simulink model "sim2"  (R2015b)
settings: Solver=VariableStepAuto  StartTime=0.0  StopTime=50  RelTol=1e-3
values from neighbouring files (symbols this model uses):
  A1 = [0 1 0 ... (first row only)    [tp2.m]
  A2 = [0 1 0 ... (first row only)    [tp2.m]
  B1 = [0 ... (first row only)    [tp2.m]
  B2 = [0 ... (first row only)    [tp2.m]
  K1 = place(A1,B1,[lmb(1) lmb(2) 0])    [tp2.m]
  K2 = place(A2,B2,[lmb(1) lmb(2) 0])    [tp2.m]
  thetaIni1 = [theta1i 0 0]    [tp2.m]
  thetaIni2 = [theta2i 0 0]    [tp2.m]
settings Model: Creator=max.Sonzogni  LastModifiedBy=max.sonzogni

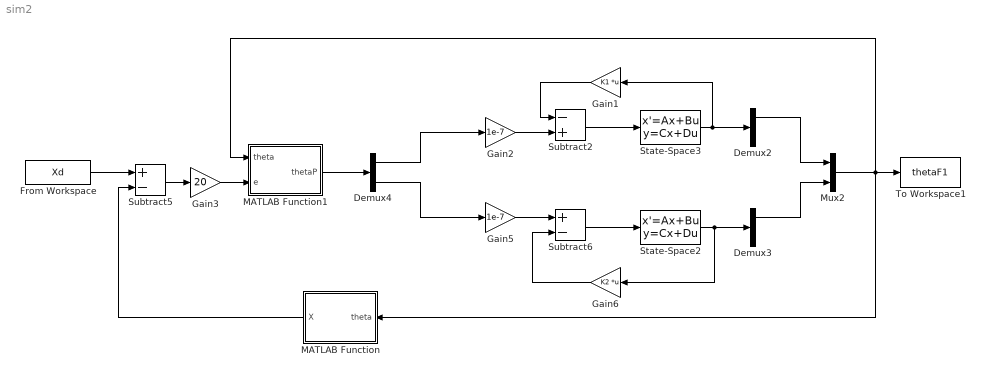
== system sim2 ==
  Demux2 : Demux  Outputs=3
  Demux3 : Demux  Outputs=3
  Demux4 : Demux  Outputs=2
  From Workspace : FromWorkspace  VariableName=Xd  SampleTime=0
  Gain1 : Gain  Gain=K1  Multiplication=Matrix(K*u)
  Gain2 : Gain  Gain=1e-7
  Gain3 : Gain  Gain=20
  Gain5 : Gain  Gain=1e-7
  Gain6 : Gain  Gain=K2  Multiplication=Matrix(K*u)
  MATLAB Function : MATLAB Function  TreatAsAtomicUnit=on
  MATLAB Function1 : MATLAB Function  TreatAsAtomicUnit=on
  Mux2 : Mux  Inputs=2
  State-Space2 : StateSpace  A=A2  B=B2  C=eye(3)  D=zeros(3,1)  X0=thetaIni2
  State-Space3 : StateSpace  A=A1  B=B1  C=eye(3)  D=zeros(3,1)  X0=thetaIni1
  Subtract2 : Sum  Inputs=-+
  Subtract5 : Sum  Inputs=+-
  Subtract6 : Sum  Inputs=+-
  To Workspace1 : ToWorkspace  VariableName=thetaF1  SampleTime=-1
  wires:
  State-Space2/1 -> Demux3/1, Gain6/1
  State-Space3/1 -> Gain1/1, Demux2/1
  Demux2/1 -> Mux2/1
  Demux3/1 -> Mux2/2
  From Workspace/1 -> Subtract5/1
  Demux4/1 -> Gain2/1
  Subtract2/1 -> State-Space3/1
  Demux4/2 -> Gain5/1
  Gain5/1 -> Subtract6/1
  Gain6/1 -> Subtract6/2
  Subtract6/1 -> State-Space2/1
  Gain2/1 -> Subtract2/2
  MATLAB Function/1(X) -> Subtract5/2
  Gain1/1 -> Subtract2/1
  MATLAB Function1/1(thetaP) -> Demux4/1
  Mux2/1 -> To Workspace1/1, MATLAB Function/1(theta), MATLAB Function1/1(theta)
  Gain3/1 -> MATLAB Function1/2(e)
  Subtract5/1 -> Gain3/1

== matlab function sim2/MATLAB Function1 ==
  data: theta input; e input; thetaP output
function thetaP = Jmoins1(theta,e)

l1 = 0.65;
l2 = 0.35;

teta = theta;

J = [-l1*sin(teta(1))-l2*sin(teta(1)+teta(2)) -l2*sin(teta(1)+teta(2))
    l1*cos(teta(1))+l2*cos(teta(1)+teta(2)) l2*cos(teta(1)+teta(2))];

J1 = inv(J);

thetaP = J1*e;

end

== matlab function sim2/MATLAB Function ==
  data: X output; theta input
function X = MGD(theta)

l1 = 0.65;
l2 = 0.35;

X = zeros(1,2);

X(1) = l1*cos(theta(1))+l2*cos(theta(1)+theta(2));
X(2) = l1*sin(theta(1))+l2*sin(theta(1)+theta(2));

end
